simulink model "rocketlqrfinal"  (R2025b)
settings: Solver=VariableStepAuto  StartTime=0.0  StopTime=10.0  RelTol=1e-3
values from neighbouring files (symbols this model uses):
  A = [0 1 0 0 ... (first row only)    [Controllerdesign.m]
  B = [1 0.1 ... (first row only)    [Controllerdesign.m]
  C = eye(4)    [Controllerdesign.m]
  D = zeros(4,2)    [Controllerdesign.m]
  Ki = Ka(:,5:6)    [Controllerdesign.m]
  Kx = Ka(:,1:4)    [Controllerdesign.m]
undefined symbols (not defined in the file or in its folder): Continuous, Time
libraries: simulink x1, ctrlSharedLib x1
settings Model: Creator=vaish  LastModifiedBy=vaish
settings DebuggingCC: UnderSpecifiedDimensionMsg=warning

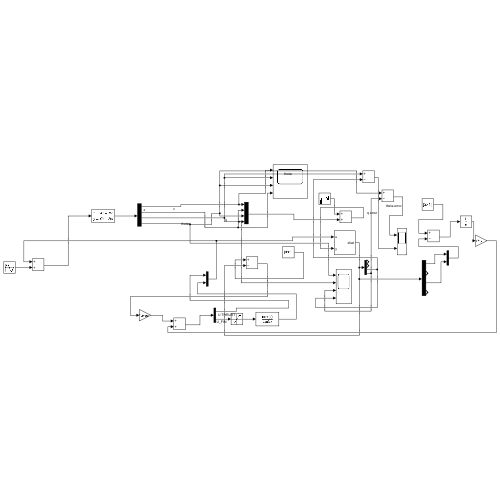
[thumbnail: Simulink's stored preview of the top-level diagram]
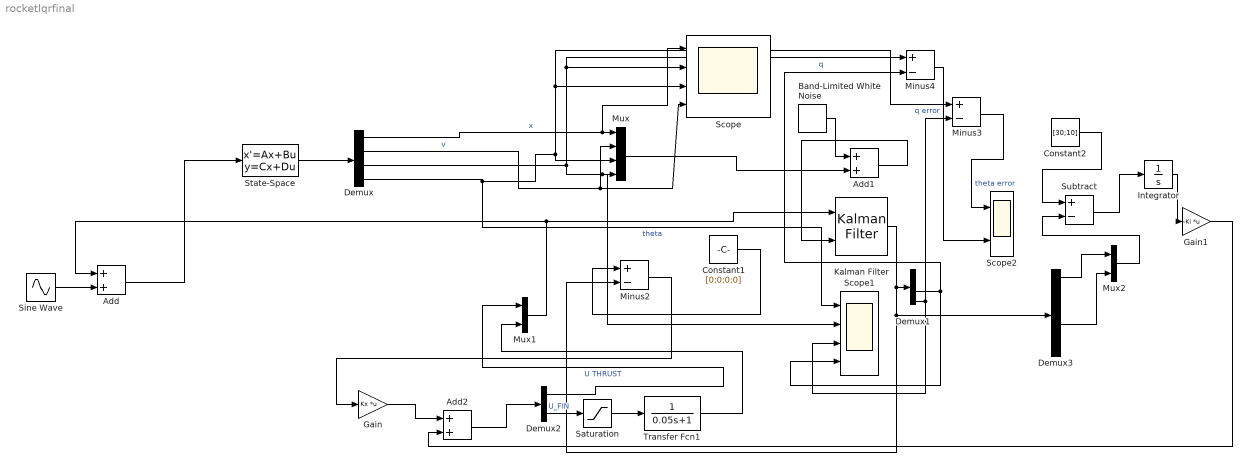
== system rocketlqrfinal ==
  Add : Sum
  Add1 : Sum
  Add2 : Sum
  Band-Limited White Noise : simulink/Sources/Band-Limited White Noise  Cov=[0.1]  Ts=0.1  seed=[23341]
  Constant1 : Constant  Value=[0;0;0;0]
  Constant2 : Constant  Value=[30;10]
  Demux : Demux
  Demux1 : Demux
  Demux2 : Demux  Outputs=2
  Demux3 : Demux
  Gain : Gain  Gain=Kx  Multiplication=Matrix(K*u) (u vector)
  Gain1 : Gain  Gain=-Ki  Multiplication=Matrix(K*u)
  Integrator : Integrator
  Kalman Filter : ctrlSharedLib/Kalman Filter  TimeDomain=Continuous-Time  UseCurrentEstimator=on  ModelSource=LTI State-Space Variable  ModelSourceVariable=sys  A=0.95  B=1  C=1  D=0  NumberOfStates=1  NumberOfInputs=1  NumberOfOutputs=1  InitialEstimateSource=Dialog  X0=0  P0=10  UseK=off  UseGH=off  NumberOfProcessNoiseInputs=1  G=1  TimeInvariantG=on  H=0  TimeInvariantH=on  Q=eye(4)  TimeInvariantQ=on  R=0.8*eye(4)  TimeInvariantR=on  N=zeros(4)  TimeInvariantN=on  AddInputPort=on  AddEnablePort=off  OutputEstimatedY=off  OutputP=off  Ts=-1
  Minus2 : Sum  Inputs=+-
  Minus3 : Sum  Inputs=+-
  Minus4 : Sum  Inputs=+-
  Mux : Mux
  Mux1 : Mux  Inputs=2
  Mux2 : Mux  Inputs=2
  Saturation : Saturate  UpperLimit=15  LowerLimit=-15
  Scope : Scope  NumInputPorts=4
      settings: ActiveDisplayYMinimum=-9.5563844639601356  ActiveDisplayYMaximum=36.999484897378629
  Scope1 : Scope  NumInputPorts=4
      settings: ActiveDisplayYMinimum=-4.9534893148616641  ActiveDisplayYMaximum=9.1543019037781761
  Scope2 : Scope  NumInputPorts=2
      settings: ActiveDisplayYMinimum=-10.939180765899067  ActiveDisplayYMaximum=13.762757464686274  DataLoggingVariableName=ScopeData2
  Sine Wave : Sin  Amplitude=2  Frequency=0.1  SampleTime=0
  State-Space : StateSpace  A=A  B=B  C=C  D=D  InitialCondition=0
  Subtract : Sum  Inputs=+-
  Transfer Fcn1 : TransferFcn  Denominator=[0.05 1]
  wires:
  State-Space/1 -> Demux/1
  Demux/2 -> Mux/2, Scope/4  "v"
  Demux/4 -> Scope1/1, Scope/3, Minus3/1, Mux/3  "theta"
  Demux/3 -> Mux/4, Scope1/2, Scope/2, Minus4/1  "q"
  Sine Wave/1 -> Add/2
  Add/1 -> State-Space/1
  Mux1/1 -> Add/1, Kalman Filter/1
  Constant1/1 -> Minus2/1
  Minus2/1 -> Gain/1
  Band-Limited White Noise/1 -> Add1/1
  Demux/1 -> Scope/1, Mux/1  "x"
  Mux/1 -> Add1/2
  Kalman Filter/1 -> Minus2/2, Demux3/1, Demux1/1
  Add1/1 -> Kalman Filter/2
  Demux1/3 -> Minus4/2, Scope1/4
  Demux1/4 -> Scope1/3, Minus3/2
  Minus3/1 -> Scope2/1  "theta error"
  Minus4/1 -> Scope2/2  "q error"
  Demux2/2 -> Saturation/1  "U_FIN"
  Transfer Fcn1/1 -> Mux1/2
  Demux2/1 -> Mux1/1  "U THRUST"
  Gain/1 -> Add2/1
  Saturation/1 -> Transfer Fcn1/1
  Demux3/1 -> Mux2/1
  Demux3/3 -> Mux2/2
  Constant2/1 -> Subtract/1
  Mux2/1 -> Subtract/2
  Subtract/1 -> Integrator/1
  Integrator/1 -> Gain1/1
  Gain1/1 -> Add2/2
  Add2/1 -> Demux2/1
